simulink model "QUESTION5"  (R2020a)
settings: Solver=VariableStepAuto  StartTime=0.0  StopTime=10.0  RelTol=1e-3
undefined symbols (not defined in the file): C, R
settings Model: Creator=anjal  LastModifiedBy=anjal

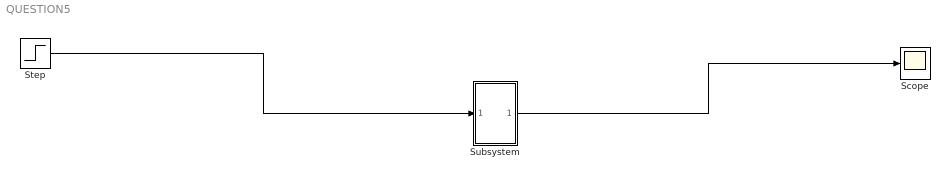
== system QUESTION5 ==
  Scope : Scope
  Step : Step  SampleTime=0
  Subsystem : Subsystem  TreatAsAtomicUnit=on
  wires:
  Step/1 -> Subsystem/1(In1)
  Subsystem/1(Out1) -> Scope/1

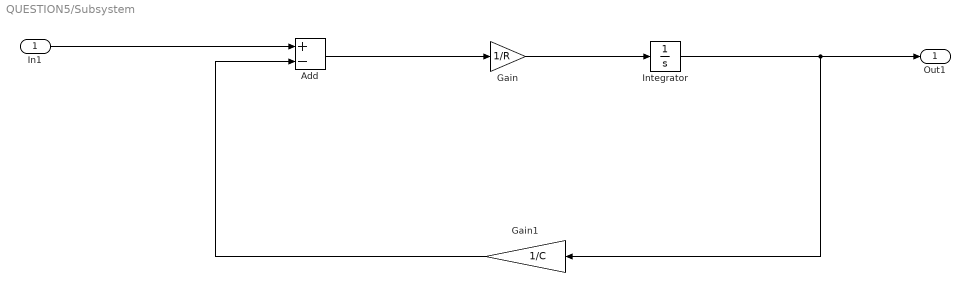
== system QUESTION5/Subsystem ==
  In1 : Inport
  Add : Sum  Inputs=+-
  Gain : Gain  Gain=1/R  LockScale=on
  Gain1 : Gain  Gain=1/C
  Integrator : Integrator
  Out1 : Outport
  wires:
  Gain/1 -> Integrator/1
  Integrator/1 -> Out1/1, Gain1/1
  In1/1 -> Add/1
  Add/1 -> Gain/1
  Gain1/1 -> Add/2
